simulink model "Harvest_DuffingCL"  (R2015a)
settings: Solver=ode4  StartTime=0.0  StopTime=tf-dt  FixedStep=dt  RelTol=1e-3
values from neighbouring files (symbols this model uses):
  chi = 0.51    [main_ETDF.m]    (also in main_OGY_R01.m = 0.05; piezomagbeam.m = phys_param(2))
  dt = 0.001    [main_ETDF.m]
  K = -1.3    [main_ETDF.m]
  k = 0.51    [main_ETDF.m]
  lam = 0.04    [main_ETDF.m]
  R = 0.95    [main_ETDF.m]
  si = 0.01    [main_ETDF.m]
  w = 0.8    [main_ETDF.m]
  x0 = [1 0 0]    [main_ETDF.m]    (also in main_OGY_R01.m = zeros(3,N_cycles))
libraries: simulink x1
settings Model: Creator=jose_  LastModifiedBy=jose_

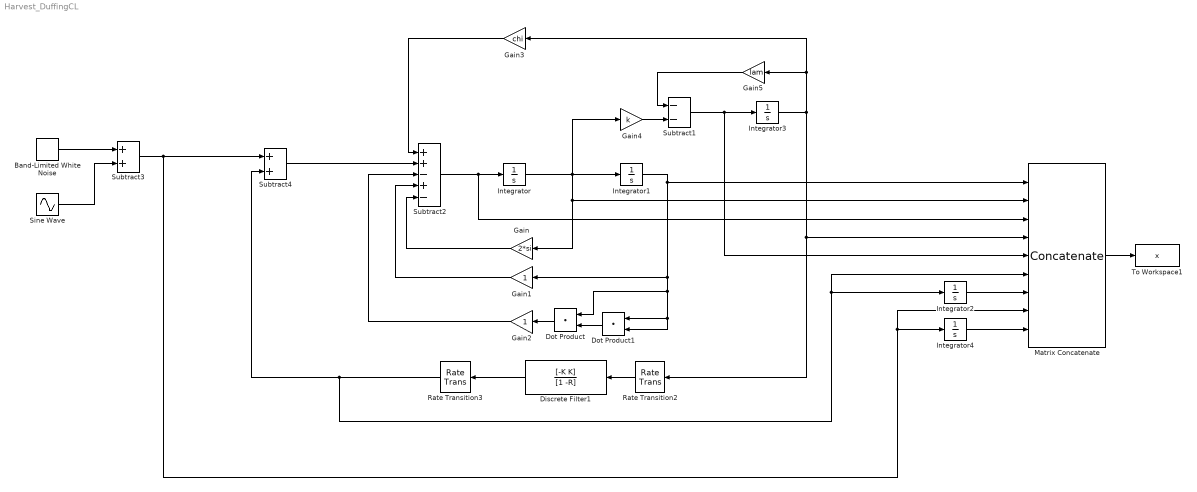
== system Harvest_DuffingCL ==
  Band-Limited White Noise : simulink/Sources/Band-Limited White Noise  Cov=[0.00]  Ts=dt  seed=[23341]
  Discrete Filter1 : DiscreteFilter  Numerator=[-K K]  Denominator=[1 -R]
  Dot Product : DotProduct  InputSameDT=on  OutDataTypeStr=Inherit: Inherit via internal rule
  Dot Product1 : DotProduct  InputSameDT=on  OutDataTypeStr=Inherit: Inherit via internal rule
  Gain : Gain  Gain=2*si
  Gain1 : Gain
  Gain2 : Gain
  Gain3 : Gain  Gain=chi
  Gain4 : Gain  Gain=k
  Gain5 : Gain  Gain=lam
  Integrator : Integrator  InitialCondition=x0(2)  ContinuousStateAttributes='Velocity'
  Integrator1 : Integrator  InitialCondition=x0(1)  ContinuousStateAttributes='Position'
  Integrator2 : Integrator
  Integrator3 : Integrator  InitialCondition=x0(3)  ContinuousStateAttributes='voltage'
  Integrator4 : Integrator
  Matrix Concatenate : Concatenate  NumInputs=9  Mode=Multidimensional array  ConcatenateDimension=2
  Rate Transition2 : RateTransition  OutPortSampleTime=T
  Rate Transition3 : RateTransition  OutPortSampleTime=dt
  Sine Wave : Sin  Amplitude=u  Frequency=w  SampleTime=dt
  Subtract1 : Sum  Inputs=--
  Subtract2 : Sum  Inputs=++-+-
  Subtract3 : Sum
  Subtract4 : Sum
  To Workspace1 : ToWorkspace  VariableName=x  SampleTime=-1
      settings: Save2DSignal=2-D array (concatenate along first dimension)
  wires:
  Subtract2/1 -> Matrix Concatenate/3, Integrator/1
  Dot Product/1 -> Gain2/1
  Dot Product1/1 -> Dot Product/2
  Subtract1/1 -> Matrix Concatenate/5, Integrator3/1
  Gain4/1 -> Subtract1/2
  Matrix Concatenate/1 -> To Workspace1/1
  Integrator1/1 -> Dot Product1/2, Dot Product1/1, Dot Product/1, Gain1/1, Matrix Concatenate/1
  Gain5/1 -> Subtract1/1
  Integrator/1 -> Integrator1/1, Gain4/1, Gain/1, Matrix Concatenate/2
  Gain3/1 -> Subtract2/1
  Gain2/1 -> Subtract2/3
  Gain1/1 -> Subtract2/4
  Gain/1 -> Subtract2/5
  Sine Wave/1 -> Subtract3/2
  Band-Limited White Noise/1 -> Subtract3/1
  Subtract4/1 -> Subtract2/2
  Integrator3/1 -> Gain3/1, Gain5/1, Matrix Concatenate/4, Rate Transition2/1
  Rate Transition2/1 -> Discrete Filter1/1
  Discrete Filter1/1 -> Rate Transition3/1
  Rate Transition3/1 -> Integrator2/1, Matrix Concatenate/6, Subtract4/2
  Subtract3/1 -> Matrix Concatenate/8, Integrator4/1, Subtract4/1
  Integrator4/1 -> Matrix Concatenate/9
  Integrator2/1 -> Matrix Concatenate/7
